simulink model "ALU_04_SS"  (R2022a)
settings: Solver=VariableStepAuto  StartTime=0.0  StopTime=10.0  RelTol=1e-3
undefined symbols (not defined in the file or in its folder): xc7z010iclg225
libraries: hdlBasic x1537, vmcUtilities x1
(part 1 of 8)
settings Model: Creator=sebas  LastModifiedBy=sebas

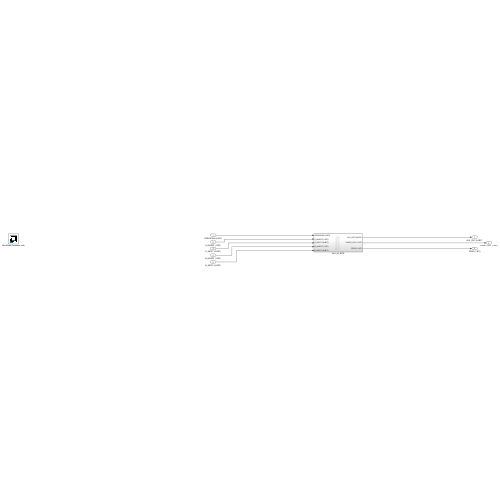
[thumbnail: Simulink's stored preview of the top-level diagram]
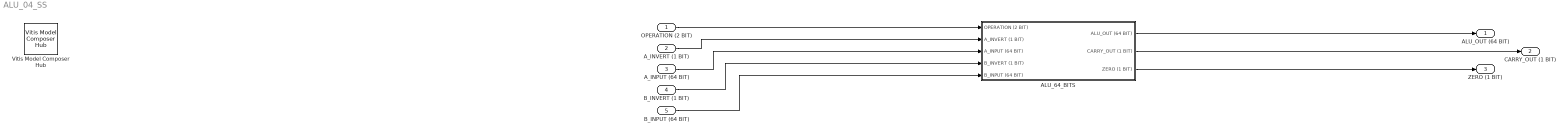
== system ALU_04_SS ==
  OPERATION (2 BIT) : Inport
  A_INVERT (1 BIT) : Inport  Port=2
  A_INPUT (64 BIT) : Inport  Port=3
  B_INVERT (1 BIT) : Inport  Port=4
  B_INPUT (64 BIT) : Inport  Port=5
  ALU_64_BITS : Subsystem
  Vitis Model Composer Hub : vmcUtilities/Vitis Model Composer Hub  Tag=genX  CodeGeneration=off  TargetDirectory=./code  ExportType=AI Engines  IpVendor=xilinx.com  IpLibrary=hls  IpVersion=1.0  IpHWLanguage=Verilog  AieCompilerOptions={}  AieSimulatorOptions={}  CreateTestbench=off  TestbenchStackSize=10  RunAieSim=off  AieSimTimeout=50000  RunAieSimProfiling=off  LaunchVitisAnalyzer=off  PlotOutput=off  RunX86Sim=off  X86SimTimeout=10  GenHwImage=off  PlatformType=Not Specified  HwSystemType=Baremetal  HwValidationTarget=hw  ProjDevice=xc7z010iclg225-1L  ProjDevicePart=xc7z010iclg225-1L  SamplePeriod=-1  ClockFrequency=200  DataPathParallelism=1  xilinxfamily=zynq  part=xc7z010i  speed=-1L  package=clg225  directory=./netlist  testbench=off  incr_netlist=off  synthesis_tool=Vivado  clock_wrapper=Clock Enables  dbl_ovrd=According to Block Masks  dcm_input_clock_period=10  sysclk_period=10  simulink_period=1  eval_field=0  LogFileName=''  NThreads=4
  ALU_OUT (64 BIT) : Outport
  CARRY_OUT (1 BIT) : Outport  Port=2
  ZERO (1 BIT) : Outport  Port=3
  wires:
  OPERATION (2 BIT)/1 -> ALU_64_BITS/1(OPERATION (2 BIT))
  A_INVERT (1 BIT)/1 -> ALU_64_BITS/2(A_INVERT (1 BIT))
  A_INPUT (64 BIT)/1 -> ALU_64_BITS/3(A_INPUT (64 BIT))
  B_INVERT (1 BIT)/1 -> ALU_64_BITS/4(B_INVERT (1 BIT))
  B_INPUT (64 BIT)/1 -> ALU_64_BITS/5(B_INPUT (64 BIT))
  ALU_64_BITS/1(ALU_OUT (64 BIT)) -> ALU_OUT (64 BIT)/1
  ALU_64_BITS/2(CARRY_OUT (1 BIT)) -> CARRY_OUT (1 BIT)/1
  ALU_64_BITS/3(ZERO (1 BIT)) -> ZERO (1 BIT)/1
